simulink model "QuadRotor_PID_Simulink3d"  (R2014a)
settings: Solver=ode45  StartTime=0.0  StopTime=inf
PreLoadFcn:
  | load CommandsBus
model workspace (MAT data in the model file):
  MCOS : class17 (value not decoded)
  MCOS : class17 (value not decoded)
undefined symbols (not defined in the file or in its folder): X, Y, Z
libraries: sm_lib x829, nesl_utility x156, simulink x12, fl_lib x4, vrlib x4, aerolibtransform2 x1
(part 2 of 18)

== system QuadRotor_PID_Simulink3d/quadSimulation/Plant_Quad_Base/Quad_Roll/Convert1 ==
  In1 : Inport
  Add : Sum  Inputs=+-
  Constant : Constant  Value=pi/2
  ConvertAngle : MATLAB Function  TreatAsAtomicUnit=on
  Out1 : Outport
  wires:
  Constant/1 -> Add/2
  Add/1 -> ConvertAngle/1(radAngle)
  In1/1 -> Add/1
  ConvertAngle/1(AngleDeg) -> Out1/1

== system QuadRotor_PID_Simulink3d/quadSimulation/Plant_Quad_Base/Quad_Roll/Convert2 ==
  In1 : Inport
  ConvertAngle : MATLAB Function  TreatAsAtomicUnit=on
  Out1 : Outport
  wires:
  In1/1 -> ConvertAngle/1(radAngle)
  ConvertAngle/1(AngleDeg) -> Out1/1

== system QuadRotor_PID_Simulink3d/quadSimulation/Plant_Quad_Base/Quad_Roll/Convert3 ==
  In1 : Inport
  Gain : Gain  Gain=-1
  Out1 : Outport
  wires:
  In1/1 -> Gain/1
  Gain/1 -> Out1/1

== system QuadRotor_PID_Simulink3d/quadSimulation/Plant_Quad_Base/Quad_Roll/QuadRotor ==
  motor_A : Inport
  motor_B : Inport  Port=2
  motor_C : Inport  Port=3
  motor_D : Inport  Port=4
  MontagemRingSuperior_1_RIGID : Subsystem
  P1 : Subsystem
  P2 : Subsystem
  P3 : Subsystem
  P4 : Subsystem
  ReferenceFrame : sm_lib/Frames and Transforms/Reference Frame  BlockFunction=simmechanics.library.frames_transforms.reference_frame
  RingInferior_1_RIGID : Subsystem
  Transform : sm_lib/Frames and Transforms/Rigid Transform  TranslationMethod=Cartesian  TranslationLengthUnit=mm  TranslationStandardAxis=+Z  TranslationStandardOffset=0  TranslationCartesianOffset=[-2.914334999999997e-16 -0.75 -2.4715275000000003e-16]  TranslationROffset=0  TranslationROffsetUnits=m  TranslationZOffset=0  TranslationZOffsetUnits=m  TranslationThetaOffset=0  TranslationThetaOffsetUnits=deg  RotationMethod=ArbitraryAxis  RotationAngleUnits=rad  RotationStandardAxis=+Z  RotationAngle=1.5707963267948963  RotationArbitraryAxis=[-1 -2.7673873760513264e-16 -7.0654160640769886e-16]  FollAlignAxisA=+X  BaseAlignAxisA=+Y  FollAlignAxisB=+Y  BaseAlignAxisB=+Z  BlockFunction=simmechanics.library.frames_transforms.rigid_transform
  Transform1 : sm_lib/Frames and Transforms/Rigid Transform  TranslationMethod=None  TranslationLengthUnit=m  TranslationStandardAxis=+Z  TranslationStandardOffset=0  TranslationCartesianOffset=[0 0 0]  TranslationROffset=0  TranslationROffsetUnits=m  TranslationZOffset=0  TranslationZOffsetUnits=m  TranslationThetaOffset=0  TranslationThetaOffsetUnits=deg  RotationMethod=None  RotationAngleUnits=deg  RotationStandardAxis=+Z  RotationAngle=0  RotationArbitraryAxis=[0 0 1]  FollAlignAxisA=+X  BaseAlignAxisA=+Y  FollAlignAxisB=+Y  BaseAlignAxisB=+Z  BlockFunction=simmechanics.library.frames_transforms.rigid_transform
  F : PMIOPort  Port=1  Side=Left
  ThrustB : Outport
  ThrustA : Outport  Port=2
  ThrustC : Outport  Port=3
  ThrustD : Outport  Port=4
  wires:
  motor_B/1 -> P1/1(SpdMotorB)
  motor_A/1 -> P2/1(SpdMotorA)
  motor_C/1 -> P3/1(SpdMotorC)
  motor_D/1 -> P4/1(SpdMotorD)
  P1/1(ThrustB) -> ThrustB/1
  P2/1(ThrustA) -> ThrustA/1
  P3/1(ThrustC) -> ThrustC/1
  P4/1(ThrustD) -> ThrustD/1
  connections:
  P2/RConn1 -- ReferenceFrame/RConn1 -- MontagemRingSuperior_1_RIGID/RConn1 -- P4/RConn1 -- P3/RConn1 -- P1/RConn1 -- Transform/LConn1 -- Transform1/LConn1
  Transform/RConn1 -- F/RConn1
  RingInferior_1_RIGID/LConn1 -- Transform1/RConn1

== system QuadRotor_PID_Simulink3d/quadSimulation/Plant_Quad_Base/Quad_Roll_Pitch_Yaw/BaseTestes ==
  BaseTestes : Subsystem
  ConnQuad : PMIOPort  Port=1  Side=Left
  Roll : Outport
  Pitch : Outport  Port=2
  Yaw : Outport  Port=3
  Altitude : Outport  Port=4
  wires:
  BaseTestes/1(Roll) -> Roll/1
  BaseTestes/2(Pitch) -> Pitch/1
  BaseTestes/3(Yaw) -> Yaw/1
  BaseTestes/4(Altitude) -> Altitude/1
  connections:
  ConnQuad/RConn1 -- BaseTestes/LConn1

== system QuadRotor_PID_Simulink3d/quadSimulation/Plant_Quad_Base/Quad_Roll_Pitch_Yaw/Convert ==
  In1 : Inport
  Add : Sum
  Constant : Constant  Value=pi/2
  ConvertAngle : MATLAB Function  TreatAsAtomicUnit=on
  Out1 : Outport
  wires:
  Constant/1 -> Add/2
  Add/1 -> ConvertAngle/1(radAngle)
  In1/1 -> Add/1
  ConvertAngle/1(AngleDeg) -> Out1/1

== system QuadRotor_PID_Simulink3d/quadSimulation/Plant_Quad_Base/Quad_Roll_Pitch_Yaw/Convert1 ==
  In1 : Inport
  Add : Sum  Inputs=+-
  Constant : Constant  Value=pi/2
  ConvertAngle : MATLAB Function  TreatAsAtomicUnit=on
  Out1 : Outport
  wires:
  Constant/1 -> Add/2
  Add/1 -> ConvertAngle/1(radAngle)
  In1/1 -> Add/1
  ConvertAngle/1(AngleDeg) -> Out1/1

== system QuadRotor_PID_Simulink3d/quadSimulation/Plant_Quad_Base/Quad_Roll_Pitch_Yaw/Convert2 ==
  In1 : Inport
  ConvertAngle : MATLAB Function  TreatAsAtomicUnit=on
  Out1 : Outport
  wires:
  In1/1 -> ConvertAngle/1(radAngle)
  ConvertAngle/1(AngleDeg) -> Out1/1

== system QuadRotor_PID_Simulink3d/quadSimulation/Plant_Quad_Base/Quad_Roll_Pitch_Yaw/Convert3 ==
  In1 : Inport
  Gain : Gain  Gain=-1
  Out1 : Outport
  wires:
  In1/1 -> Gain/1
  Gain/1 -> Out1/1

== system QuadRotor_PID_Simulink3d/quadSimulation/Plant_Quad_Base/Quad_Roll_Pitch_Yaw/QuadRotor ==
  motor_A : Inport
  motor_B : Inport  Port=2
  motor_C : Inport  Port=3
  motor_D : Inport  Port=4
  MontagemRingSuperior_1_RIGID : Subsystem
  P1 : Subsystem
  P2 : Subsystem
  P3 : Subsystem
  P4 : Subsystem
  ReferenceFrame : sm_lib/Frames and Transforms/Reference Frame  BlockFunction=simmechanics.library.frames_transforms.reference_frame
  RingInferior_1_RIGID : Subsystem
  Transform : sm_lib/Frames and Transforms/Rigid Transform  TranslationMethod=Cartesian  TranslationLengthUnit=mm  TranslationStandardAxis=+Z  TranslationStandardOffset=0  TranslationCartesianOffset=[-2.914334999999997e-16 -0.75 -2.4715275000000003e-16]  TranslationROffset=0  TranslationROffsetUnits=m  TranslationZOffset=0  TranslationZOffsetUnits=m  TranslationThetaOffset=0  TranslationThetaOffsetUnits=deg  RotationMethod=ArbitraryAxis  RotationAngleUnits=rad  RotationStandardAxis=+Z  RotationAngle=1.5707963267948963  RotationArbitraryAxis=[-1 -2.7673873760513264e-16 -7.0654160640769886e-16]  FollAlignAxisA=+X  BaseAlignAxisA=+Y  FollAlignAxisB=+Y  BaseAlignAxisB=+Z  BlockFunction=simmechanics.library.frames_transforms.rigid_transform
  Transform1 : sm_lib/Frames and Transforms/Rigid Transform  TranslationMethod=None  TranslationLengthUnit=m  TranslationStandardAxis=+Z  TranslationStandardOffset=0  TranslationCartesianOffset=[0 0 0]  TranslationROffset=0  TranslationROffsetUnits=m  TranslationZOffset=0  TranslationZOffsetUnits=m  TranslationThetaOffset=0  TranslationThetaOffsetUnits=deg  RotationMethod=None  RotationAngleUnits=deg  RotationStandardAxis=+Z  RotationAngle=0  RotationArbitraryAxis=[0 0 1]  FollAlignAxisA=+X  BaseAlignAxisA=+Y  FollAlignAxisB=+Y  BaseAlignAxisB=+Z  BlockFunction=simmechanics.library.frames_transforms.rigid_transform
  F : PMIOPort  Port=1  Side=Left
  ThrustB : Outport
  ThrustA : Outport  Port=2
  ThrustC : Outport  Port=3
  ThrustD : Outport  Port=4
  wires:
  motor_B/1 -> P1/1(SpdMotorB)
  motor_A/1 -> P2/1(SpdMotorA)
  motor_C/1 -> P3/1(SpdMotorC)
  motor_D/1 -> P4/1(SpdMotorD)
  P1/1(ThrustB) -> ThrustB/1
  P2/1(ThrustA) -> ThrustA/1
  P3/1(ThrustC) -> ThrustC/1
  P4/1(ThrustD) -> ThrustD/1
  connections:
  P2/RConn1 -- ReferenceFrame/RConn1 -- MontagemRingSuperior_1_RIGID/RConn1 -- P4/RConn1 -- P3/RConn1 -- P1/RConn1 -- Transform/LConn1 -- Transform1/LConn1
  Transform/RConn1 -- F/RConn1
  RingInferior_1_RIGID/LConn1 -- Transform1/RConn1

== system QuadRotor_PID_Simulink3d/quadSimulation/Plant_Quad_Base/Quad_Roll_Pitch_Yaw_Altitude/BaseTestes ==
  BaseTestes : Subsystem
  ConnQuad : PMIOPort  Port=1  Side=Left
  Roll : Outport
  Pitch : Outport  Port=2
  Yaw : Outport  Port=3
  Altitude : Outport  Port=4
  wires:
  BaseTestes/1(Roll) -> Roll/1
  BaseTestes/2(Pitch) -> Pitch/1
  BaseTestes/3(Yaw) -> Yaw/1
  BaseTestes/4(Altitude) -> Altitude/1
  connections:
  ConnQuad/RConn1 -- BaseTestes/LConn1

== system QuadRotor_PID_Simulink3d/quadSimulation/Plant_Quad_Base/Quad_Roll_Pitch_Yaw_Altitude/Convert ==
  In1 : Inport
  Add : Sum
  Constant : Constant  Value=pi/2
  ConvertAngle : MATLAB Function  TreatAsAtomicUnit=on
  Out1 : Outport
  wires:
  Constant/1 -> Add/2
  Add/1 -> ConvertAngle/1(radAngle)
  In1/1 -> Add/1
  ConvertAngle/1(AngleDeg) -> Out1/1

== system QuadRotor_PID_Simulink3d/quadSimulation/Plant_Quad_Base/Quad_Roll_Pitch_Yaw_Altitude/Convert1 ==
  In1 : Inport
  Add : Sum  Inputs=+-
  Constant : Constant  Value=pi/2
  ConvertAngle : MATLAB Function  TreatAsAtomicUnit=on
  Out1 : Outport
  wires:
  Constant/1 -> Add/2
  Add/1 -> ConvertAngle/1(radAngle)
  In1/1 -> Add/1
  ConvertAngle/1(AngleDeg) -> Out1/1

== system QuadRotor_PID_Simulink3d/quadSimulation/Plant_Quad_Base/Quad_Roll_Pitch_Yaw_Altitude/Convert2 ==
  In1 : Inport
  ConvertAngle : MATLAB Function  TreatAsAtomicUnit=on
  Out1 : Outport
  wires:
  In1/1 -> ConvertAngle/1(radAngle)
  ConvertAngle/1(AngleDeg) -> Out1/1

== system QuadRotor_PID_Simulink3d/quadSimulation/Plant_Quad_Base/Quad_Roll_Pitch_Yaw_Altitude/Convert3 ==
  In1 : Inport
  Gain : Gain  Gain=-1
  Out1 : Outport
  wires:
  In1/1 -> Gain/1
  Gain/1 -> Out1/1

== system QuadRotor_PID_Simulink3d/quadSimulation/Plant_Quad_Base/Quad_Roll_Pitch_Yaw_Altitude/QuadRotor ==
  motor_A : Inport
  motor_B : Inport  Port=2
  motor_C : Inport  Port=3
  motor_D : Inport  Port=4
  MontagemRingSuperior_1_RIGID : Subsystem
  P1 : Subsystem
  P2 : Subsystem
  P3 : Subsystem
  P4 : Subsystem
  ReferenceFrame : sm_lib/Frames and Transforms/Reference Frame  BlockFunction=simmechanics.library.frames_transforms.reference_frame
  RingInferior_1_RIGID : Subsystem
  Transform : sm_lib/Frames and Transforms/Rigid Transform  TranslationMethod=Cartesian  TranslationLengthUnit=mm  TranslationStandardAxis=+Z  TranslationStandardOffset=0  TranslationCartesianOffset=[-2.914334999999997e-16 -0.75 -2.4715275000000003e-16]  TranslationROffset=0  TranslationROffsetUnits=m  TranslationZOffset=0  TranslationZOffsetUnits=m  TranslationThetaOffset=0  TranslationThetaOffsetUnits=deg  RotationMethod=ArbitraryAxis  RotationAngleUnits=rad  RotationStandardAxis=+Z  RotationAngle=1.5707963267948963  RotationArbitraryAxis=[-1 -2.7673873760513264e-16 -7.0654160640769886e-16]  FollAlignAxisA=+X  BaseAlignAxisA=+Y  FollAlignAxisB=+Y  BaseAlignAxisB=+Z  BlockFunction=simmechanics.library.frames_transforms.rigid_transform
  Transform1 : sm_lib/Frames and Transforms/Rigid Transform  TranslationMethod=None  TranslationLengthUnit=m  TranslationStandardAxis=+Z  TranslationStandardOffset=0  TranslationCartesianOffset=[0 0 0]  TranslationROffset=0  TranslationROffsetUnits=m  TranslationZOffset=0  TranslationZOffsetUnits=m  TranslationThetaOffset=0  TranslationThetaOffsetUnits=deg  RotationMethod=None  RotationAngleUnits=deg  RotationStandardAxis=+Z  RotationAngle=0  RotationArbitraryAxis=[0 0 1]  FollAlignAxisA=+X  BaseAlignAxisA=+Y  FollAlignAxisB=+Y  BaseAlignAxisB=+Z  BlockFunction=simmechanics.library.frames_transforms.rigid_transform
  F : PMIOPort  Port=1  Side=Left
  ThrustB : Outport
  ThrustA : Outport  Port=2
  ThrustC : Outport  Port=3
  ThrustD : Outport  Port=4
  wires:
  motor_B/1 -> P1/1(SpdMotorB)
  motor_A/1 -> P2/1(SpdMotorA)
  motor_C/1 -> P3/1(SpdMotorC)
  motor_D/1 -> P4/1(SpdMotorD)
  P1/1(ThrustB) -> ThrustB/1
  P2/1(ThrustA) -> ThrustA/1
  P3/1(ThrustC) -> ThrustC/1
  P4/1(ThrustD) -> ThrustD/1
  connections:
  P2/RConn1 -- ReferenceFrame/RConn1 -- MontagemRingSuperior_1_RIGID/RConn1 -- P4/RConn1 -- P3/RConn1 -- P1/RConn1 -- Transform/LConn1 -- Transform1/LConn1
  Transform/RConn1 -- F/RConn1
  RingInferior_1_RIGID/LConn1 -- Transform1/RConn1

== system QuadRotor_PID_Simulink3d/quadSimulation/Plant_Quad_Base/Quad_Yaw/BaseTestes ==
  BaseTestes : Subsystem
  ConnQuad : PMIOPort  Port=1  Side=Left
  Roll : Outport
  Pitch : Outport  Port=2
  Yaw : Outport  Port=3
  Altitude : Outport  Port=4
  wires:
  BaseTestes/1(Roll) -> Roll/1
  BaseTestes/2(Pitch) -> Pitch/1
  BaseTestes/3(Yaw) -> Yaw/1
  BaseTestes/4(Altitude) -> Altitude/1
  connections:
  ConnQuad/RConn1 -- BaseTestes/LConn1

== system QuadRotor_PID_Simulink3d/quadSimulation/Plant_Quad_Base/Quad_Yaw/Convert ==
  In1 : Inport
  Add : Sum
  Constant : Constant  Value=pi/2
  ConvertAngle : MATLAB Function  TreatAsAtomicUnit=on
  Out1 : Outport
  wires:
  Constant/1 -> Add/2
  Add/1 -> ConvertAngle/1(radAngle)
  In1/1 -> Add/1
  ConvertAngle/1(AngleDeg) -> Out1/1

== system QuadRotor_PID_Simulink3d/quadSimulation/Plant_Quad_Base/Quad_Yaw/Convert1 ==
  In1 : Inport
  Add : Sum  Inputs=+-
  Constant : Constant  Value=pi/2
  ConvertAngle : MATLAB Function  TreatAsAtomicUnit=on
  Out1 : Outport
  wires:
  Constant/1 -> Add/2
  Add/1 -> ConvertAngle/1(radAngle)
  In1/1 -> Add/1
  ConvertAngle/1(AngleDeg) -> Out1/1

== system QuadRotor_PID_Simulink3d/quadSimulation/Plant_Quad_Base/Quad_Yaw/Convert2 ==
  In1 : Inport
  ConvertAngle : MATLAB Function  TreatAsAtomicUnit=on
  Out1 : Outport
  wires:
  In1/1 -> ConvertAngle/1(radAngle)
  ConvertAngle/1(AngleDeg) -> Out1/1

== system QuadRotor_PID_Simulink3d/quadSimulation/Plant_Quad_Base/Quad_Yaw/Convert3 ==
  In1 : Inport
  Gain : Gain  Gain=-1
  Out1 : Outport
  wires:
  In1/1 -> Gain/1
  Gain/1 -> Out1/1

== system QuadRotor_PID_Simulink3d/quadSimulation/Plant_Quad_Base/Quad_Yaw/QuadRotor ==
  motor_A : Inport
  motor_B : Inport  Port=2
  motor_C : Inport  Port=3
  motor_D : Inport  Port=4
  MontagemRingSuperior_1_RIGID : Subsystem
  P1 : Subsystem
  P2 : Subsystem
  P3 : Subsystem
  P4 : Subsystem
  ReferenceFrame : sm_lib/Frames and Transforms/Reference Frame  BlockFunction=simmechanics.library.frames_transforms.reference_frame
  RingInferior_1_RIGID : Subsystem
  Transform : sm_lib/Frames and Transforms/Rigid Transform  TranslationMethod=Cartesian  TranslationLengthUnit=mm  TranslationStandardAxis=+Z  TranslationStandardOffset=0  TranslationCartesianOffset=[-2.914334999999997e-16 -0.75 -2.4715275000000003e-16]  TranslationROffset=0  TranslationROffsetUnits=m  TranslationZOffset=0  TranslationZOffsetUnits=m  TranslationThetaOffset=0  TranslationThetaOffsetUnits=deg  RotationMethod=ArbitraryAxis  RotationAngleUnits=rad  RotationStandardAxis=+Z  RotationAngle=1.5707963267948963  RotationArbitraryAxis=[-1 -2.7673873760513264e-16 -7.0654160640769886e-16]  FollAlignAxisA=+X  BaseAlignAxisA=+Y  FollAlignAxisB=+Y  BaseAlignAxisB=+Z  BlockFunction=simmechanics.library.frames_transforms.rigid_transform
  Transform1 : sm_lib/Frames and Transforms/Rigid Transform  TranslationMethod=None  TranslationLengthUnit=m  TranslationStandardAxis=+Z  TranslationStandardOffset=0  TranslationCartesianOffset=[0 0 0]  TranslationROffset=0  TranslationROffsetUnits=m  TranslationZOffset=0  TranslationZOffsetUnits=m  TranslationThetaOffset=0  TranslationThetaOffsetUnits=deg  RotationMethod=None  RotationAngleUnits=deg  RotationStandardAxis=+Z  RotationAngle=0  RotationArbitraryAxis=[0 0 1]  FollAlignAxisA=+X  BaseAlignAxisA=+Y  FollAlignAxisB=+Y  BaseAlignAxisB=+Z  BlockFunction=simmechanics.library.frames_transforms.rigid_transform
  F : PMIOPort  Port=1  Side=Left
  ThrustB : Outport
  ThrustA : Outport  Port=2
  ThrustC : Outport  Port=3
  ThrustD : Outport  Port=4
  wires:
  motor_B/1 -> P1/1(SpdMotorB)
  motor_A/1 -> P2/1(SpdMotorA)
  motor_C/1 -> P3/1(SpdMotorC)
  motor_D/1 -> P4/1(SpdMotorD)
  P1/1(ThrustB) -> ThrustB/1
  P2/1(ThrustA) -> ThrustA/1
  P3/1(ThrustC) -> ThrustC/1
  P4/1(ThrustD) -> ThrustD/1
  connections:
  P2/RConn1 -- ReferenceFrame/RConn1 -- MontagemRingSuperior_1_RIGID/RConn1 -- P4/RConn1 -- P3/RConn1 -- P1/RConn1 -- Transform/LConn1 -- Transform1/LConn1
  Transform/RConn1 -- F/RConn1
  RingInferior_1_RIGID/LConn1 -- Transform1/RConn1

== system QuadRotor_PID_Simulink3d/quadSimulation/Plant_Quad_Base/Quad_Yaw_Altitude/BaseTestes ==
  BaseTestes : Subsystem
  ConnQuad : PMIOPort  Port=1  Side=Left
  Roll : Outport
  Pitch : Outport  Port=2
  Yaw : Outport  Port=3
  Altitude : Outport  Port=4
  wires:
  BaseTestes/1(Roll) -> Roll/1
  BaseTestes/2(Pitch) -> Pitch/1
  BaseTestes/3(Yaw) -> Yaw/1
  BaseTestes/4(Altitude) -> Altitude/1
  connections:
  ConnQuad/RConn1 -- BaseTestes/LConn1

== system QuadRotor_PID_Simulink3d/quadSimulation/Plant_Quad_Base/Quad_Yaw_Altitude/Convert ==
  In1 : Inport
  Add : Sum
  Constant : Constant  Value=pi/2
  ConvertAngle : MATLAB Function  TreatAsAtomicUnit=on
  Out1 : Outport
  wires:
  Constant/1 -> Add/2
  Add/1 -> ConvertAngle/1(radAngle)
  In1/1 -> Add/1
  ConvertAngle/1(AngleDeg) -> Out1/1

== system QuadRotor_PID_Simulink3d/quadSimulation/Plant_Quad_Base/Quad_Yaw_Altitude/Convert1 ==
  In1 : Inport
  Add : Sum  Inputs=+-
  Constant : Constant  Value=pi/2
  ConvertAngle : MATLAB Function  TreatAsAtomicUnit=on
  Out1 : Outport
  wires:
  Constant/1 -> Add/2
  Add/1 -> ConvertAngle/1(radAngle)
  In1/1 -> Add/1
  ConvertAngle/1(AngleDeg) -> Out1/1

== system QuadRotor_PID_Simulink3d/quadSimulation/Plant_Quad_Base/Quad_Yaw_Altitude/Convert2 ==
  In1 : Inport
  ConvertAngle : MATLAB Function  TreatAsAtomicUnit=on
  Out1 : Outport
  wires:
  In1/1 -> ConvertAngle/1(radAngle)
  ConvertAngle/1(AngleDeg) -> Out1/1

== system QuadRotor_PID_Simulink3d/quadSimulation/Plant_Quad_Base/Quad_Yaw_Altitude/Convert3 ==
  In1 : Inport
  Gain : Gain  Gain=-1
  Out1 : Outport
  wires:
  In1/1 -> Gain/1
  Gain/1 -> Out1/1

== system QuadRotor_PID_Simulink3d/quadSimulation/Plant_Quad_Base/Quad_Yaw_Altitude/QuadRotor ==
  motor_A : Inport
  motor_B : Inport  Port=2
  motor_C : Inport  Port=3
  motor_D : Inport  Port=4
  MontagemRingSuperior_1_RIGID : Subsystem
  P1 : Subsystem
  P2 : Subsystem
  P3 : Subsystem
  P4 : Subsystem
  ReferenceFrame : sm_lib/Frames and Transforms/Reference Frame  BlockFunction=simmechanics.library.frames_transforms.reference_frame
  RingInferior_1_RIGID : Subsystem
  Transform : sm_lib/Frames and Transforms/Rigid Transform  TranslationMethod=Cartesian  TranslationLengthUnit=mm  TranslationStandardAxis=+Z  TranslationStandardOffset=0  TranslationCartesianOffset=[-2.914334999999997e-16 -0.75 -2.4715275000000003e-16]  TranslationROffset=0  TranslationROffsetUnits=m  TranslationZOffset=0  TranslationZOffsetUnits=m  TranslationThetaOffset=0  TranslationThetaOffsetUnits=deg  RotationMethod=ArbitraryAxis  RotationAngleUnits=rad  RotationStandardAxis=+Z  RotationAngle=1.5707963267948963  RotationArbitraryAxis=[-1 -2.7673873760513264e-16 -7.0654160640769886e-16]  FollAlignAxisA=+X  BaseAlignAxisA=+Y  FollAlignAxisB=+Y  BaseAlignAxisB=+Z  BlockFunction=simmechanics.library.frames_transforms.rigid_transform
  Transform1 : sm_lib/Frames and Transforms/Rigid Transform  TranslationMethod=None  TranslationLengthUnit=m  TranslationStandardAxis=+Z  TranslationStandardOffset=0  TranslationCartesianOffset=[0 0 0]  TranslationROffset=0  TranslationROffsetUnits=m  TranslationZOffset=0  TranslationZOffsetUnits=m  TranslationThetaOffset=0  TranslationThetaOffsetUnits=deg  RotationMethod=None  RotationAngleUnits=deg  RotationStandardAxis=+Z  RotationAngle=0  RotationArbitraryAxis=[0 0 1]  FollAlignAxisA=+X  BaseAlignAxisA=+Y  FollAlignAxisB=+Y  BaseAlignAxisB=+Z  BlockFunction=simmechanics.library.frames_transforms.rigid_transform
  F : PMIOPort  Port=1  Side=Left
  ThrustB : Outport
  ThrustA : Outport  Port=2
  ThrustC : Outport  Port=3
  ThrustD : Outport  Port=4
  wires:
  motor_B/1 -> P1/1(SpdMotorB)
  motor_A/1 -> P2/1(SpdMotorA)
  motor_C/1 -> P3/1(SpdMotorC)
  motor_D/1 -> P4/1(SpdMotorD)
  P1/1(ThrustB) -> ThrustB/1
  P2/1(ThrustA) -> ThrustA/1
  P3/1(ThrustC) -> ThrustC/1
  P4/1(ThrustD) -> ThrustD/1
  connections:
  P2/RConn1 -- ReferenceFrame/RConn1 -- MontagemRingSuperior_1_RIGID/RConn1 -- P4/RConn1 -- P3/RConn1 -- P1/RConn1 -- Transform/LConn1 -- Transform1/LConn1
  Transform/RConn1 -- F/RConn1
  RingInferior_1_RIGID/LConn1 -- Transform1/RConn1

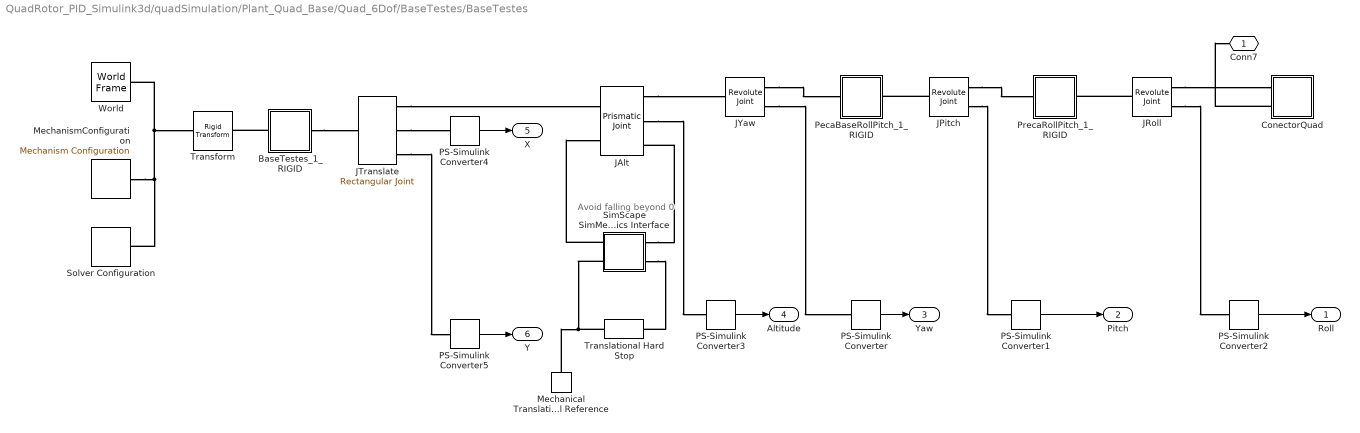
== system QuadRotor_PID_Simulink3d/quadSimulation/Plant_Quad_Base/Quad_6Dof/BaseTestes/BaseTestes ==
  note: Avoid falling beyond 0
  BaseTestes_1_RIGID : Subsystem
  ConectorQuad : Subsystem
  JAlt : sm_lib/Joints/Prismatic Joint  SenseConstraintForce=off  SenseConstraintForceX=off  SenseConstraintForceY=off  SenseConstraintForceZ=off  SenseConstraintTorque=off  SenseConstraintTorqueX=off  SenseConstraintTorqueY=off  SenseConstraintTorqueZ=off  SenseTotalForce=off  SenseTotalForceX=off  SenseTotalForceY=off  SenseTotalForceZ=off  SenseTotalTorque=off  SenseTotalTorqueX=off  SenseTotalTorqueY=off  SenseTotalTorqueZ=off  CompositeWrenchDir=FollowerOnBase  CompositeWrenchFrame=BaseFrame  EquilibriumPosition=0  EquilibriumPositionUnits=m  SpringStiffness=0  SpringStiffnessUnits=N/m  DampingCoefficient=0  DampingCoefficientUnits=N/(m/s)  TorqueActuationMode=InputTorque  MotionActuationMode=ComputedMotion  SensePosition=on  SenseVelocity=on  SenseAcceleration=off  SenseTorqueForce=off  PositionTargetValue=0  PositionTargetValueUnits=m  PositionTargetSpecify=off  PositionTargetPriority=High  VelocityTargetValue=0  VelocityTargetValueUnits=m/s  VelocityTargetSpecify=off  VelocityTargetPriority=High  BlockFunction=simmechanics.library.joints.prismatic_joint
  JPitch : sm_lib/Joints/Revolute Joint  SenseConstraintForce=off  SenseConstraintForceX=off  SenseConstraintForceY=off  SenseConstraintForceZ=off  SenseConstraintTorque=off  SenseConstraintTorqueX=off  SenseConstraintTorqueY=off  SenseConstraintTorqueZ=off  SenseTotalForce=off  SenseTotalForceX=off  SenseTotalForceY=off  SenseTotalForceZ=off  SenseTotalTorque=off  SenseTotalTorqueX=off  SenseTotalTorqueY=off  SenseTotalTorqueZ=off  CompositeWrenchDir=FollowerOnBase  CompositeWrenchFrame=BaseFrame  EquilibriumPosition=0  EquilibriumPositionUnits=rad  SpringStiffness=0  SpringStiffnessUnits=m*N/rad  DampingCoefficient=0.001  DampingCoefficientUnits=m*s*N/rad  TorqueActuationMode=NoTorque  MotionActuationMode=ComputedMotion  SensePosition=on  SenseVelocity=off  SenseAcceleration=off  SenseTorqueForce=off  PositionTargetValue=90  PositionTargetValueUnits=deg  PositionTargetSpecify=on  PositionTargetPriority=Low  VelocityTargetValue=0  VelocityTargetValueUnits=deg/s  VelocityTargetSpecify=off  VelocityTargetPriority=High  BlockFunction=simmechanics.library.joints.revolute_joint
  JRoll : sm_lib/Joints/Revolute Joint  SenseConstraintForce=off  SenseConstraintForceX=off  SenseConstraintForceY=off  SenseConstraintForceZ=off  SenseConstraintTorque=off  SenseConstraintTorqueX=off  SenseConstraintTorqueY=off  SenseConstraintTorqueZ=off  SenseTotalForce=off  SenseTotalForceX=off  SenseTotalForceY=off  SenseTotalForceZ=off  SenseTotalTorque=off  SenseTotalTorqueX=off  SenseTotalTorqueY=off  SenseTotalTorqueZ=off  CompositeWrenchDir=FollowerOnBase  CompositeWrenchFrame=BaseFrame  EquilibriumPosition=0  EquilibriumPositionUnits=rad  SpringStiffness=0  SpringStiffnessUnits=m*N/rad  DampingCoefficient=0.001  DampingCoefficientUnits=m*s*N/rad  TorqueActuationMode=NoTorque  MotionActuationMode=ComputedMotion  SensePosition=on  SenseVelocity=off  SenseAcceleration=off  SenseTorqueForce=off  PositionTargetValue=-90  PositionTargetValueUnits=deg  PositionTargetSpecify=on  PositionTargetPriority=Low  VelocityTargetValue=0  VelocityTargetValueUnits=deg/s  VelocityTargetSpecify=off  VelocityTargetPriority=High  BlockFunction=simmechanics.library.joints.revolute_joint
  JTranslate : sm_lib/Joints/Rectangular Joint  SenseConstraintForce=off  SenseConstraintForceX=off  SenseConstraintForceY=off  SenseConstraintForceZ=off  SenseConstraintTorque=off  SenseConstraintTorqueX=off  SenseConstraintTorqueY=off  SenseConstraintTorqueZ=off  SenseTotalForce=off  SenseTotalForceX=off  SenseTotalForceY=off  SenseTotalForceZ=off  SenseTotalTorque=off  SenseTotalTorqueX=off  SenseTotalTorqueY=off  SenseTotalTorqueZ=off  CompositeWrenchDir=FollowerOnBase  CompositeWrenchFrame=BaseFrame  PxEquilibriumPosition=0  PxEquilibriumPositionUnits=m  PxSpringStiffness=0  PxSpringStiffnessUnits=N/m  PxDampingCoefficient=0  PxDampingCoefficientUnits=N/(m/s)  PxTorqueActuationMode=NoTorque  PxMotionActuationMode=ComputedMotion  PxSensePosition=on  PxSenseVelocity=off  PxSenseAcceleration=off  PxSenseTorqueForce=off  PxPositionTargetValue=0  PxPositionTargetValueUnits=m  PxPositionTargetSpecify=off  PxPositionTargetPriority=High  PxVelocityTargetValue=0  PxVelocityTargetValueUnits=m/s  PxVelocityTargetSpecify=off  PxVelocityTargetPriority=High  PyEquilibriumPosition=0  PyEquilibriumPositionUnits=m  PySpringStiffness=0  PySpringStiffnessUnits=N/m  PyDampingCoefficient=0  PyDampingCoefficientUnits=N/(m/s)  PyTorqueActuationMode=NoTorque  PyMotionActuationMode=ComputedMotion  PySensePosition=on  PySenseVelocity=off  PySenseAcceleration=off  PySenseTorqueForce=off  PyPositionTargetValue=0  PyPositionTargetValueUnits=m  PyPositionTargetSpecify=off  PyPositionTargetPriority=High  PyVelocityTargetValue=0  PyVelocityTargetValueUnits=m/s  PyVelocityTargetSpecify=off  PyVelocityTargetPriority=High  BlockFunction=simmechanics.library.joints.rectangular_joint
  JYaw : sm_lib/Joints/Revolute Joint  SenseConstraintForce=off  SenseConstraintForceX=off  SenseConstraintForceY=off  SenseConstraintForceZ=off  SenseConstraintTorque=off  SenseConstraintTorqueX=off  SenseConstraintTorqueY=off  SenseConstraintTorqueZ=off  SenseTotalForce=off  SenseTotalForceX=off  SenseTotalForceY=off  SenseTotalForceZ=off  SenseTotalTorque=off  SenseTotalTorqueX=off  SenseTotalTorqueY=off  SenseTotalTorqueZ=off  CompositeWrenchDir=FollowerOnBase  CompositeWrenchFrame=BaseFrame  EquilibriumPosition=0  EquilibriumPositionUnits=rad  SpringStiffness=0  SpringStiffnessUnits=m*N/rad  DampingCoefficient=0.001  DampingCoefficientUnits=m*s*N/rad  TorqueActuationMode=NoTorque  MotionActuationMode=ComputedMotion  SensePosition=on  SenseVelocity=off  SenseAcceleration=off  SenseTorqueForce=off  PositionTargetValue=0  PositionTargetValueUnits=deg  PositionTargetSpecify=on  PositionTargetPriority=Low  VelocityTargetValue=0  VelocityTargetValueUnits=deg/s  VelocityTargetSpecify=off  VelocityTargetPriority=High  BlockFunction=simmechanics.library.joints.revolute_joint
  Mechanical Translational Reference : fl_lib/Mechanical/Translational Elements/Mechanical Translational Reference
  MechanismConfiguration : sm_lib/Utilities/Mechanism Configuration  UniformGravity=Constant  GravityVector=[0 -9.81 0]  GravityUnits=m/s^2  LinearizationDelta=0.001  BlockFunction=simmechanics.library.utilities.mechanism_configuration
  PS-Simulink Converter{,1,3..5} (5 alike) : nesl_utility/PS-Simulink Converter  PhysicalDomain=network_engine_domain  SubClassName=ps_output  LeftPortType=input  RightPortType=output  PseudoPeriodic=off  Frequencies=[]  Unit=1  AffineConversion=off
  PS-Simulink Converter2 : nesl_utility/PS-Simulink Converter  PhysicalDomain=network_engine_domain  SubClassName=ps_output  LeftPortType=input  RightPortType=output  PseudoPeriodic=off  Frequencies=[]  Unit=rad  AffineConversion=off
  PecaBaseRollPitch_1_RIGID : Subsystem
  PrecaRollPitch_1_RIGID : Subsystem
  SimScape SimMechanics Interface : Subsystem
  Solver Configuration : nesl_utility/Solver Configuration  PhysicalDomain=network_engine_domain  SubClassName=solver  LeftPortType=input  RightPortType=generic  Accelerate=off  Tones=[]  Harmonics=[]  SimulateNoise=off  Profile=off  UseLocalSampling=off  EnableSwitchedLinearOptims=on  FrequencyDomain=off  UseCCode=off  RelTol=0.001  AbsTol=1e-06  MinStep=1e-09  ToWorkspace=off  DoDC=off  ResidualTolerance=1e-09  UseLocalSolver=off  LocalSolverChoice=NE_BACKWARD_EULER_ADVANCER  LocalSolverSampleTime=0.001  DoFixedCost=off  MaxNonlinIter=3  MaxModeIter=2  LinearAlgebra=Sparse  DelaysMemoryBudget=1024  AutomaticFiltering=on  FilteringTimeConstant=0.001
  Transform : sm_lib/Frames and Transforms/Rigid Transform  TranslationMethod=None  TranslationLengthUnit=m  TranslationStandardAxis=+Z  TranslationStandardOffset=0  TranslationCartesianOffset=[0 0 0]  TranslationROffset=0  TranslationROffsetUnits=m  TranslationZOffset=0  TranslationZOffsetUnits=m  TranslationThetaOffset=0  TranslationThetaOffsetUnits=deg  RotationMethod=None  RotationAngleUnits=deg  RotationStandardAxis=+Z  RotationAngle=0  RotationArbitraryAxis=[0 0 1]  FollAlignAxisA=+X  BaseAlignAxisA=+Y  FollAlignAxisB=+Y  BaseAlignAxisB=+Z  BlockFunction=simmechanics.library.frames_transforms.rigid_transform
  Translational Hard Stop : fl_lib/Mechanical/Translational Elements/Translational Hard Stop  upper_bnd=10 m  lower_bnd=0 m  stiff_up=1e6 N/m  stiff_low=1e5 N/m  D_up=150 N/(m/s)  D_low=150 N/(m/s)  v_specify=off  v_priority=High  v=0 m/s  f_specify=off  f_priority=High  f=0 N  x_specify=on  x_priority=High  x=0 m
  World : sm_lib/Frames and Transforms/World Frame  BlockFunction=simmechanics.library.frames_transforms.world_frame
  Conn7 : PMIOPort  Port=1  Side=Left
  Roll : Outport
  Pitch : Outport  Port=2
  Yaw : Outport  Port=3
  Altitude : Outport  Port=4
  X : Outport  Port=5
  Y : Outport  Port=6
  wires:
  PS-Simulink Converter1/1 -> Pitch/1
  PS-Simulink Converter/1 -> Yaw/1
  PS-Simulink Converter2/1 -> Roll/1
  PS-Simulink Converter3/1 -> Altitude/1
  PS-Simulink Converter4/1 -> X/1
  PS-Simulink Converter5/1 -> Y/1
  connections:
  JAlt/RConn1 -- JYaw/LConn1
  ConectorQuad/LConn2 -- Conn7/RConn1
  JYaw/RConn1 -- PecaBaseRollPitch_1_RIGID/LConn1
  JPitch/LConn1 -- PecaBaseRollPitch_1_RIGID/RConn1
  JPitch/RConn1 -- PrecaRollPitch_1_RIGID/LConn1
  JRoll/LConn1 -- PrecaRollPitch_1_RIGID/RConn1
  BaseTestes_1_RIGID/LConn1 -- Transform/RConn1
  JRoll/RConn1 -- ConectorQuad/LConn1
  JRoll/RConn2 -- PS-Simulink Converter2/LConn1
  JYaw/RConn2 -- PS-Simulink Converter/LConn1
  JPitch/RConn2 -- PS-Simulink Converter1/LConn1
  MechanismConfiguration/RConn1 -- Solver Configuration/RConn1 -- World/RConn1 -- Transform/LConn1
  JAlt/RConn2 -- PS-Simulink Converter3/LConn1
  JTranslate/RConn1 -- JAlt/LConn1
  JTranslate/RConn2 -- PS-Simulink Converter4/LConn1
  JTranslate/RConn3 -- PS-Simulink Converter5/LConn1
  BaseTestes_1_RIGID/RConn1 -- JTranslate/LConn1
  Mechanical Translational Reference/LConn1 -- SimScape SimMechanics Interface/LConn2 -- Translational Hard Stop/LConn1
  SimScape SimMechanics Interface/LConn1 -- JAlt/LConn2
  SimScape SimMechanics Interface/RConn2 -- Translational Hard Stop/RConn1
  SimScape SimMechanics Interface/RConn1 -- JAlt/RConn3

== system QuadRotor_PID_Simulink3d/quadSimulation/Plant_Quad_Base/Quad_6Dof/QuadRotor/MontagemRingSuperior_1_RIGID ==
  ReferenceFrame : sm_lib/Frames and Transforms/Reference Frame  BlockFunction=simmechanics.library.frames_transforms.reference_frame
  RingTopo_1_RIGID : Subsystem
  Transform : sm_lib/Frames and Transforms/Rigid Transform  TranslationMethod=Cartesian  TranslationLengthUnit=mm  TranslationStandardAxis=+Z  TranslationStandardOffset=0  TranslationCartesianOffset=[-37.365400000000001 -6.2970799999999993 0]  TranslationROffset=0  TranslationROffsetUnits=m  TranslationZOffset=0  TranslationZOffsetUnits=m  TranslationThetaOffset=0  TranslationThetaOffsetUnits=deg  RotationMethod=None  RotationAngleUnits=deg  RotationStandardAxis=+Z  RotationAngle=0  RotationArbitraryAxis=[0 0 1]  FollAlignAxisA=+X  BaseAlignAxisA=+Y  FollAlignAxisB=+Y  BaseAlignAxisB=+Z  BlockFunction=simmechanics.library.frames_transforms.rigid_transform
  Transform1 : sm_lib/Frames and Transforms/Rigid Transform  TranslationMethod=Cartesian  TranslationLengthUnit=mm  TranslationStandardAxis=+Z  TranslationStandardOffset=0  TranslationCartesianOffset=[-37.365400000000001 40.7971 -6.5503199999999999e-12]  TranslationROffset=0  TranslationROffsetUnits=m  TranslationZOffset=0  TranslationZOffsetUnits=m  TranslationThetaOffset=0  TranslationThetaOffsetUnits=deg  RotationMethod=ArbitraryAxis  RotationAngleUnits=rad  RotationStandardAxis=+Z  RotationAngle=3.1415926535897012  RotationArbitraryAxis=[0 1 0]  FollAlignAxisA=+X  BaseAlignAxisA=+Y  FollAlignAxisB=+Y  BaseAlignAxisB=+Z  BlockFunction=simmechanics.library.frames_transforms.rigid_transform
  F : PMIOPort  Port=1  Side=Right
  connections:
  RingTopo_1_RIGID/LConn1 -- Transform/RConn1
  Transform/LConn1 -- ReferenceFrame/RConn1 -- Transform1/RConn1
  Transform1/LConn1 -- F/RConn1

== system QuadRotor_PID_Simulink3d/quadSimulation/Plant_Quad_Base/Quad_6Dof/QuadRotor/P1 ==
  SpdMotorB : Inport
  MotorB : Subsystem
  PernaInferior_1_RIGID : Subsystem
  PernaSuperior_1_RIGID : Subsystem
  ReferenceFrame : sm_lib/Frames and Transforms/Reference Frame  BlockFunction=simmechanics.library.frames_transforms.reference_frame
  Transform : sm_lib/Frames and Transforms/Rigid Transform  TranslationMethod=Cartesian  TranslationLengthUnit=mm  TranslationStandardAxis=+Z  TranslationStandardOffset=0  TranslationCartesianOffset=[36.732399999999998 2.09903 0]  TranslationROffset=0  TranslationROffsetUnits=m  TranslationZOffset=0  TranslationZOffsetUnits=m  TranslationThetaOffset=0  TranslationThetaOffsetUnits=deg  RotationMethod=None  RotationAngleUnits=deg  RotationStandardAxis=+Z  RotationAngle=0  RotationArbitraryAxis=[0 0 1]  FollAlignAxisA=+X  BaseAlignAxisA=+Y  FollAlignAxisB=+Y  BaseAlignAxisB=+Z  BlockFunction=simmechanics.library.frames_transforms.rigid_transform
  Transform1 : sm_lib/Frames and Transforms/Rigid Transform  TranslationMethod=Cartesian  TranslationLengthUnit=mm  TranslationStandardAxis=+Z  TranslationStandardOffset=0  TranslationCartesianOffset=[36.732399999999998 13.599 0]  TranslationROffset=0  TranslationROffsetUnits=m  TranslationZOffset=0  TranslationZOffsetUnits=m  TranslationThetaOffset=0  TranslationThetaOffsetUnits=deg  RotationMethod=ArbitraryAxis  RotationAngleUnits=rad  RotationStandardAxis=+Z  RotationAngle=3.1415926535897931  RotationArbitraryAxis=[1 0 0]  FollAlignAxisA=+X  BaseAlignAxisA=+Y  FollAlignAxisB=+Y  BaseAlignAxisB=+Z  BlockFunction=simmechanics.library.frames_transforms.rigid_transform
  Transform2 : sm_lib/Frames and Transforms/Rigid Transform  TranslationMethod=Cartesian  TranslationLengthUnit=mm  TranslationStandardAxis=+Z  TranslationStandardOffset=0  TranslationCartesianOffset=[0 9.4009699999999992 -36.732399999999998]  TranslationROffset=0  TranslationROffsetUnits=m  TranslationZOffset=0  TranslationZOffsetUnits=m  TranslationThetaOffset=0  TranslationThetaOffsetUnits=deg  RotationMethod=ArbitraryAxis  RotationAngleUnits=rad  RotationStandardAxis=+Z  RotationAngle=1.5707963267948974  RotationArbitraryAxis=[-0 -1 -0]  FollAlignAxisA=+X  BaseAlignAxisA=+Y  FollAlignAxisB=+Y  BaseAlignAxisB=+Z  BlockFunction=simmechanics.library.frames_transforms.rigid_transform
  F : PMIOPort  Port=1  Side=Right
  ThrustB : Outport
  wires:
  SpdMotorB/1 -> MotorB/1(SpdMotor)
  MotorB/1(ThrustDebug) -> ThrustB/1
  connections:
  PernaInferior_1_RIGID/LConn1 -- Transform/RConn1
  PernaSuperior_1_RIGID/LConn1 -- Transform1/RConn1
  ReferenceFrame/RConn1 -- MotorB/LConn1 -- Transform/LConn1 -- Transform1/LConn1 -- Transform2/RConn1
  Transform2/LConn1 -- F/RConn1

== system QuadRotor_PID_Simulink3d/quadSimulation/Plant_Quad_Base/Quad_6Dof/QuadRotor/P2 ==
  SpdMotorA : Inport
  MotorA : Subsystem
  PernaInferior_1_RIGID : Subsystem
  PernaSuperior_1_RIGID : Subsystem
  ReferenceFrame : sm_lib/Frames and Transforms/Reference Frame  BlockFunction=simmechanics.library.frames_transforms.reference_frame
  Transform : sm_lib/Frames and Transforms/Rigid Transform  TranslationMethod=Cartesian  TranslationLengthUnit=mm  TranslationStandardAxis=+Z  TranslationStandardOffset=0  TranslationCartesianOffset=[36.732399999999998 2.09903 0]  TranslationROffset=0  TranslationROffsetUnits=m  TranslationZOffset=0  TranslationZOffsetUnits=m  TranslationThetaOffset=0  TranslationThetaOffsetUnits=deg  RotationMethod=None  RotationAngleUnits=deg  RotationStandardAxis=+Z  RotationAngle=0  RotationArbitraryAxis=[0 0 1]  FollAlignAxisA=+X  BaseAlignAxisA=+Y  FollAlignAxisB=+Y  BaseAlignAxisB=+Z  BlockFunction=simmechanics.library.frames_transforms.rigid_transform
  Transform1 : sm_lib/Frames and Transforms/Rigid Transform  TranslationMethod=Cartesian  TranslationLengthUnit=mm  TranslationStandardAxis=+Z  TranslationStandardOffset=0  TranslationCartesianOffset=[36.732399999999998 13.599 0]  TranslationROffset=0  TranslationROffsetUnits=m  TranslationZOffset=0  TranslationZOffsetUnits=m  TranslationThetaOffset=0  TranslationThetaOffsetUnits=deg  RotationMethod=ArbitraryAxis  RotationAngleUnits=rad  RotationStandardAxis=+Z  RotationAngle=3.1415926535897931  RotationArbitraryAxis=[1 0 0]  FollAlignAxisA=+X  BaseAlignAxisA=+Y  FollAlignAxisB=+Y  BaseAlignAxisB=+Z  BlockFunction=simmechanics.library.frames_transforms.rigid_transform
  Transform2 : sm_lib/Frames and Transforms/Rigid Transform  TranslationMethod=Cartesian  TranslationLengthUnit=mm  TranslationStandardAxis=+Z  TranslationStandardOffset=0  TranslationCartesianOffset=[36.732399999999998 9.4009699999999992 0]  TranslationROffset=0  TranslationROffsetUnits=m  TranslationZOffset=0  TranslationZOffsetUnits=m  TranslationThetaOffset=0  TranslationThetaOffsetUnits=deg  RotationMethod=ArbitraryAxis  RotationAngleUnits=rad  RotationStandardAxis=+Z  RotationAngle=3.1415926535897927  RotationArbitraryAxis=[0 1 0]  FollAlignAxisA=+X  BaseAlignAxisA=+Y  FollAlignAxisB=+Y  BaseAlignAxisB=+Z  BlockFunction=simmechanics.library.frames_transforms.rigid_transform
  F : PMIOPort  Port=1  Side=Right
  ThrustA : Outport
  wires:
  SpdMotorA/1 -> MotorA/1(SpdMotor)
  MotorA/1(ThrustDebug) -> ThrustA/1
  connections:
  PernaInferior_1_RIGID/LConn1 -- Transform/RConn1
  PernaSuperior_1_RIGID/LConn1 -- Transform1/RConn1
  ReferenceFrame/RConn1 -- MotorA/LConn1 -- Transform/LConn1 -- Transform1/LConn1 -- Transform2/RConn1
  Transform2/LConn1 -- F/RConn1

== system QuadRotor_PID_Simulink3d/quadSimulation/Plant_Quad_Base/Quad_6Dof/QuadRotor/P3 ==
  SpdMotorC : Inport
  MotorC : Subsystem
  PernaInferior_1_RIGID : Subsystem
  PernaSuperior_1_RIGID : Subsystem
  ReferenceFrame : sm_lib/Frames and Transforms/Reference Frame  BlockFunction=simmechanics.library.frames_transforms.reference_frame
  Transform : sm_lib/Frames and Transforms/Rigid Transform  TranslationMethod=Cartesian  TranslationLengthUnit=mm  TranslationStandardAxis=+Z  TranslationStandardOffset=0  TranslationCartesianOffset=[36.732399999999998 2.09903 0]  TranslationROffset=0  TranslationROffsetUnits=m  TranslationZOffset=0  TranslationZOffsetUnits=m  TranslationThetaOffset=0  TranslationThetaOffsetUnits=deg  RotationMethod=None  RotationAngleUnits=deg  RotationStandardAxis=+Z  RotationAngle=0  RotationArbitraryAxis=[0 0 1]  FollAlignAxisA=+X  BaseAlignAxisA=+Y  FollAlignAxisB=+Y  BaseAlignAxisB=+Z  BlockFunction=simmechanics.library.frames_transforms.rigid_transform
  Transform1 : sm_lib/Frames and Transforms/Rigid Transform  TranslationMethod=Cartesian  TranslationLengthUnit=mm  TranslationStandardAxis=+Z  TranslationStandardOffset=0  TranslationCartesianOffset=[36.732399999999998 13.599 0]  TranslationROffset=0  TranslationROffsetUnits=m  TranslationZOffset=0  TranslationZOffsetUnits=m  TranslationThetaOffset=0  TranslationThetaOffsetUnits=deg  RotationMethod=ArbitraryAxis  RotationAngleUnits=rad  RotationStandardAxis=+Z  RotationAngle=3.1415926535897931  RotationArbitraryAxis=[1 0 0]  FollAlignAxisA=+X  BaseAlignAxisA=+Y  FollAlignAxisB=+Y  BaseAlignAxisB=+Z  BlockFunction=simmechanics.library.frames_transforms.rigid_transform
  Transform2 : sm_lib/Frames and Transforms/Rigid Transform  TranslationMethod=Cartesian  TranslationLengthUnit=mm  TranslationStandardAxis=+Z  TranslationStandardOffset=0  TranslationCartesianOffset=[-36.732399999999998 9.4009699999999992 0]  TranslationROffset=0  TranslationROffsetUnits=m  TranslationZOffset=0  TranslationZOffsetUnits=m  TranslationThetaOffset=0  TranslationThetaOffsetUnits=deg  RotationMethod=None  RotationAngleUnits=deg  RotationStandardAxis=+Z  RotationAngle=0  RotationArbitraryAxis=[0 0 1]  FollAlignAxisA=+X  BaseAlignAxisA=+Y  FollAlignAxisB=+Y  BaseAlignAxisB=+Z  BlockFunction=simmechanics.library.frames_transforms.rigid_transform
  F : PMIOPort  Port=1  Side=Right
  ThrustC : Outport
  wires:
  SpdMotorC/1 -> MotorC/1(SpdMotor)
  MotorC/1(ThrustDebug) -> ThrustC/1
  connections:
  PernaInferior_1_RIGID/LConn1 -- Transform/RConn1
  PernaSuperior_1_RIGID/LConn1 -- Transform1/RConn1
  ReferenceFrame/RConn1 -- MotorC/LConn1 -- Transform/LConn1 -- Transform1/LConn1 -- Transform2/RConn1
  Transform2/LConn1 -- F/RConn1

== system QuadRotor_PID_Simulink3d/quadSimulation/Plant_Quad_Base/Quad_6Dof/QuadRotor/P4 ==
  SpdMotorD : Inport
  MotorD : Subsystem
  PernaInferior_1_RIGID : Subsystem
  PernaSuperior_1_RIGID : Subsystem
  ReferenceFrame : sm_lib/Frames and Transforms/Reference Frame  BlockFunction=simmechanics.library.frames_transforms.reference_frame
  Transform : sm_lib/Frames and Transforms/Rigid Transform  TranslationMethod=Cartesian  TranslationLengthUnit=mm  TranslationStandardAxis=+Z  TranslationStandardOffset=0  TranslationCartesianOffset=[36.732399999999998 2.09903 0]  TranslationROffset=0  TranslationROffsetUnits=m  TranslationZOffset=0  TranslationZOffsetUnits=m  TranslationThetaOffset=0  TranslationThetaOffsetUnits=deg  RotationMethod=None  RotationAngleUnits=deg  RotationStandardAxis=+Z  RotationAngle=0  RotationArbitraryAxis=[0 0 1]  FollAlignAxisA=+X  BaseAlignAxisA=+Y  FollAlignAxisB=+Y  BaseAlignAxisB=+Z  BlockFunction=simmechanics.library.frames_transforms.rigid_transform
  Transform1 : sm_lib/Frames and Transforms/Rigid Transform  TranslationMethod=Cartesian  TranslationLengthUnit=mm  TranslationStandardAxis=+Z  TranslationStandardOffset=0  TranslationCartesianOffset=[36.732399999999998 13.599 0]  TranslationROffset=0  TranslationROffsetUnits=m  TranslationZOffset=0  TranslationZOffsetUnits=m  TranslationThetaOffset=0  TranslationThetaOffsetUnits=deg  RotationMethod=ArbitraryAxis  RotationAngleUnits=rad  RotationStandardAxis=+Z  RotationAngle=3.1415926535897931  RotationArbitraryAxis=[1 0 0]  FollAlignAxisA=+X  BaseAlignAxisA=+Y  FollAlignAxisB=+Y  BaseAlignAxisB=+Z  BlockFunction=simmechanics.library.frames_transforms.rigid_transform
  Transform2 : sm_lib/Frames and Transforms/Rigid Transform  TranslationMethod=Cartesian  TranslationLengthUnit=mm  TranslationStandardAxis=+Z  TranslationStandardOffset=0  TranslationCartesianOffset=[0 9.4009699999999992 36.732399999999998]  TranslationROffset=0  TranslationROffsetUnits=m  TranslationZOffset=0  TranslationZOffsetUnits=m  TranslationThetaOffset=0  TranslationThetaOffsetUnits=deg  RotationMethod=ArbitraryAxis  RotationAngleUnits=rad  RotationStandardAxis=+Z  RotationAngle=1.5707963267948954  RotationArbitraryAxis=[3.5905750000000007e-16 1 -2.9520499999999993e-17]  FollAlignAxisA=+X  BaseAlignAxisA=+Y  FollAlignAxisB=+Y  BaseAlignAxisB=+Z  BlockFunction=simmechanics.library.frames_transforms.rigid_transform
  F : PMIOPort  Port=1  Side=Right
  ThrustD : Outport
  wires:
  SpdMotorD/1 -> MotorD/1(SpdMotor)
  MotorD/1(ThrustDebug) -> ThrustD/1
  connections:
  PernaInferior_1_RIGID/LConn1 -- Transform/RConn1
  PernaSuperior_1_RIGID/LConn1 -- Transform1/RConn1
  ReferenceFrame/RConn1 -- MotorD/LConn1 -- Transform/LConn1 -- Transform1/LConn1 -- Transform2/RConn1
  Transform2/LConn1 -- F/RConn1

== system QuadRotor_PID_Simulink3d/quadSimulation/Plant_Quad_Base/Quad_6Dof/QuadRotor/RingInferior_1_RIGID ==
  ReferenceFrame : sm_lib/Frames and Transforms/Reference Frame  BlockFunction=simmechanics.library.frames_transforms.reference_frame
  Solid : sm_lib/Body Elements/Solid  InertiaType=Custom  Mass=0.1075427999999999997  MassUnits=kg  CenterOfMass=[0 1.8936499999999998 -1.3495699999999999e-12]  CenterOfMassUnits=mm  MomentsOfInertia=[4.4661399999999993 8.77881 4.4661399999999993]  MomentsOfInertiaUnits=kg*mm^2  ProductsOfInertia=[0 0 0]  ProductsOfInertiaUnits=kg*mm^2  DensityBased=on  Density=1000  DensityUnits=kg/(m^3)  GraphicType=FromGeometry  MarkerShape=Sphere  MarkerSize=10  MarkerSizeUnits=m  GraphicVisPropType=SimpleVisualProperties  GraphicDiffuseColor=[0.294118 0.294118 0.294118]  GraphicSpecularColor=[0.5 0.5 0.5 1.0]  GraphicAmbientColor=[0.15 0.15 0.15 1.0]  GraphicEmissiveColor=[0.0 0.0 0.0 1.0]  GraphicShininess=75  GraphicOpacity=1  GeometryShape=FromFile  RectangleSize=[1 1]  RectangleSizeUnits=m  BrickDimensions=[1 1 1]  BrickDimensionUnits=m  CylinderRadius=1  CylinderRadiusUnits=m  CylinderLength=1  CylinderLengthUnits=m  SphereRadius=1  SphereRadiusUnits=m  EllipsoidRadii=[1 1 1]  EllipsoidRadiiUnits=m  ExtrusionCrossSection=[1 1; -1 1; -1 -1; 1 -1]  ExtrusionCrossSectionUnits=m  ExtrusionLength=1  ExtrusionLengthUnits=m  PolygonNumSides=3  PolygonOuterRadius=1  PolygonOuterRadiusUnits=m  ExtGeomFileType=STL  ExtGeomFileName=RingInferior_Valor predeterminado_sldprt.STL  ExtGeomFileUnits=mm  RevolutionCrossSection=[1 1; 1 -1; 2 -1; 2 1]  RevolutionCrossSectionUnits=m  RevolutionExtent=Full  RevolutionAngle=180  RevolutionAngleUnits=deg  BlockFunction=simmechanics.library.body_elements.solid
  F : PMIOPort  Port=1  Side=Left
  connections:
  Solid/RConn1 -- ReferenceFrame/RConn1 -- F/RConn1
